simulink model "zhi_xian_er_jie_dao_li_bai"  (R2024a)
settings: Solver=VariableStepAuto  StartTime=0.0  StopTime=10.0  RelTol=1e-3
values from neighbouring files (symbols this model uses):
  epsilon = 100    [Parameters_SecondOrder_daolibai.m]
  k1 = 31.6228    [Parameters_SecondOrder_daolibai.m]
  K12 = 3/2 *(-2*m1-4*m2-4*m3)*g/((-4*m1-3*m2-12*m3)*l1)    (= 34.1214574899)    [Parameters_SecondOrder_daolibai.m]
  K12n = 3/2 *(-2*m1n-4*m2n-4*m3n)*g/((-4*m1n-3*m2n-12*m3n)*l1n)    (= 51.1821862348)    [Parameters_SecondOrder_daolibai.m]
  K13 = 9/2 * (m2*g)/((-4*m1-3*m2-12*m3)*l1)    (= -1.19028340081)    [Parameters_SecondOrder_daolibai.m]
  K13n = 9/2 * (m2n*g)/((-4*m1n-3*m2n-12*m3n)*l1n)    (= -1.78542510121)    [Parameters_SecondOrder_daolibai.m]
  K17 = 3/2*(-2*m1-m2-4*m3)/((-4*m1-3*m2-12*m3)*l1)    (= 3.36032388664)    [Parameters_SecondOrder_daolibai.m]
  K17n = 3/2*(-2*m1n-m2n-4*m3n)/((-4*m1n-3*m2n-12*m3n)*l1n)    (= 5.04048582996)    [Parameters_SecondOrder_daolibai.m]
  k2 = 200.8741    [Parameters_SecondOrder_daolibai.m]
  K22 = 2*g*(m1+2*(m2+m3))/(4*m2*l2-16/9*l2*(m1+3*(m2+m3)))    (= -63.9777327935)    [Parameters_SecondOrder_daolibai.m]
  K22n = 2*g*(m1n+2*(m2n+m3n))/(4*m2n*l2n-16/9*l2n*(m1n+3*(m2n+m3n)))    (= -76.7732793522)    [Parameters_SecondOrder_daolibai.m]
  K23 = -4/3*g*(m1+3*(m2+m3))/(4*m2*l2-16/9*l2*(m1+3*(m2+m3)))    (= 63.4817813765)    [Parameters_SecondOrder_daolibai.m]
  K23n = -4/3*g*(m1n+3*(m2n+m3n))/(4*m2n*l2n-16/9*l2n*(m1n+3*(m2n+m3n)))    (= 76.1781376518)    [Parameters_SecondOrder_daolibai.m]
  K27 = (2*(m1+2*(m2+m3))-4/3*(m1+3*(m2+m3)))/(4*m2*l2-16/9*l2*(m1+3*(m2+m3)))    (= -0.0506072874494)    [Parameters_SecondOrder_daolibai.m]
  K27n = (2*(m1n+2*(m2n+m3n))-4/3*(m1n+3*(m2n+m3n)))/(4*m2n*l2n-16/9*l2n*(m1n+3*(m2n+m3n)))    (= -0.0607287449393)    [Parameters_SecondOrder_daolibai.m]
  k3 = -315.0325    [Parameters_SecondOrder_daolibai.m]
  k4 = 28.4588    [Parameters_SecondOrder_daolibai.m]
  k5 = 3.6153    [Parameters_SecondOrder_daolibai.m]
  k6 = -36.2950    (= -36.295)    [Parameters_SecondOrder_daolibai.m]
  k_epsilon = 1    [Parameters_SecondOrder_daolibai.m]
  k_k = 1    [Parameters_SecondOrder_daolibai.m]
  k_mici = 1    [Parameters_SecondOrder_daolibai.m]
  Kd1_STC = 1    [Parameters_SecondOrder_daolibai.m]
  Kd2_STC = 1    [Parameters_SecondOrder_daolibai.m]
  u_down_limit = -200    [Parameters_SecondOrder_daolibai.m]
  u_up_limit = 200    [Parameters_SecondOrder_daolibai.m]
  x1_init = 1    [Parameters_SecondOrder_daolibai.m]
  x1_ref = 1.5    [Parameters_SecondOrder_daolibai.m]
  x2_init = 1    [Parameters_SecondOrder_daolibai.m]
  x2_ref = 0    [Parameters_SecondOrder_daolibai.m]
  x3_init = 1    [Parameters_SecondOrder_daolibai.m]
  x3_ref = 0    [Parameters_SecondOrder_daolibai.m]
  x4_init = 1    [Parameters_SecondOrder_daolibai.m]
  x5_init = 1    [Parameters_SecondOrder_daolibai.m]
  x6_init = 1    [Parameters_SecondOrder_daolibai.m]
settings Model: Creator=XieXW  LastModifiedBy=XieXW
settings SolverCC: ZeroCrossAlgorithm=Adaptive
settings DataIOCC: Refine=3
settings DebuggingCC: IgnoredZcDiagnostic=none

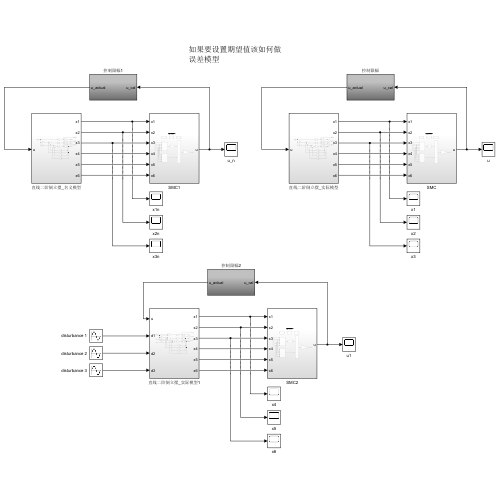
[thumbnail: Simulink's stored preview of the top-level diagram]
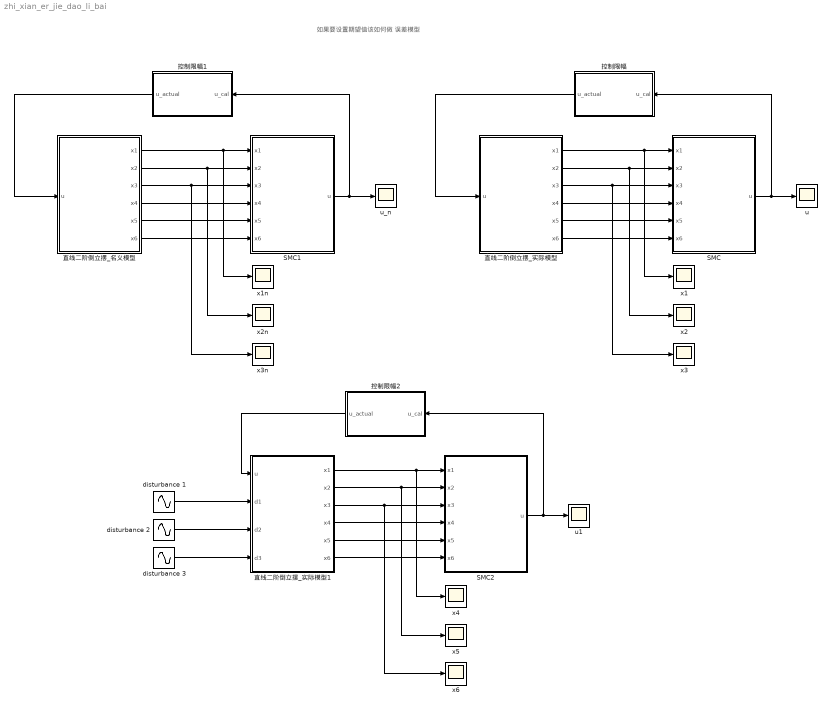
== system zhi_xian_er_jie_dao_li_bai ==
  note: 如果要设置期望值该如何做
      | 误差模型
  SMC : Subsystem
  SMC1 : Subsystem
  SMC2 : Subsystem
  disturbance 1 : Sin  Amplitude=0.05  Bias=0.1  Frequency=10  SampleTime=0
  disturbance 2 : Sin  Amplitude=0.003  Bias=0.1  Frequency=7  SampleTime=0
  disturbance 3 : Sin  Amplitude=0  Frequency=0  SampleTime=0
  u : Scope
  u1 : Scope
  u_n : Scope
  x{1..6} (6 alike) : Scope
  x1n : Scope
  x2n : Scope
  x3n : Scope
  控制限幅 : Subsystem
  控制限幅1 : Subsystem
  控制限幅2 : Subsystem
  直线二阶倒立摆_名义模型 : Subsystem
  直线二阶倒立摆_实际模型 : Subsystem
  直线二阶倒立摆_实际模型1 : Subsystem
  wires:
  直线二阶倒立摆_实际模型/1(x1) -> x1/1, SMC/1(x1)
  直线二阶倒立摆_实际模型/2(x2) -> x2/1, SMC/2(x2)
  直线二阶倒立摆_实际模型/3(x3) -> x3/1, SMC/3(x3)
  直线二阶倒立摆_实际模型/4(x4) -> SMC/4(x4)
  直线二阶倒立摆_实际模型/5(x5) -> SMC/5(x5)
  直线二阶倒立摆_实际模型/6(x6) -> SMC/6(x6)
  SMC/1(u) -> u/1, 控制限幅/1(u_cal)
  控制限幅/1(u_actual) -> 直线二阶倒立摆_实际模型/1(u)
  直线二阶倒立摆_名义模型/3(x3) -> x3n/1, SMC1/3(x3)
  SMC1/1(u) -> u_n/1, 控制限幅1/1(u_cal)
  直线二阶倒立摆_名义模型/2(x2) -> x2n/1, SMC1/2(x2)
  直线二阶倒立摆_名义模型/6(x6) -> SMC1/6(x6)
  直线二阶倒立摆_名义模型/1(x1) -> x1n/1, SMC1/1(x1)
  直线二阶倒立摆_名义模型/4(x4) -> SMC1/4(x4)
  直线二阶倒立摆_名义模型/5(x5) -> SMC1/5(x5)
  控制限幅1/1(u_actual) -> 直线二阶倒立摆_名义模型/1(u)
  直线二阶倒立摆_实际模型1/3(x3) -> x6/1, SMC2/3(x3)
  SMC2/1(u) -> u1/1, 控制限幅2/1(u_cal)
  直线二阶倒立摆_实际模型1/2(x2) -> x5/1, SMC2/2(x2)
  直线二阶倒立摆_实际模型1/6(x6) -> SMC2/6(x6)
  直线二阶倒立摆_实际模型1/1(x1) -> x4/1, SMC2/1(x1)
  直线二阶倒立摆_实际模型1/4(x4) -> SMC2/4(x4)
  直线二阶倒立摆_实际模型1/5(x5) -> SMC2/5(x5)
  控制限幅2/1(u_actual) -> 直线二阶倒立摆_实际模型1/1(u)
  disturbance 1/1 -> 直线二阶倒立摆_实际模型1/2(d1)
  disturbance 2/1 -> 直线二阶倒立摆_实际模型1/3(d2)
  disturbance 3/1 -> 直线二阶倒立摆_实际模型1/4(d3)

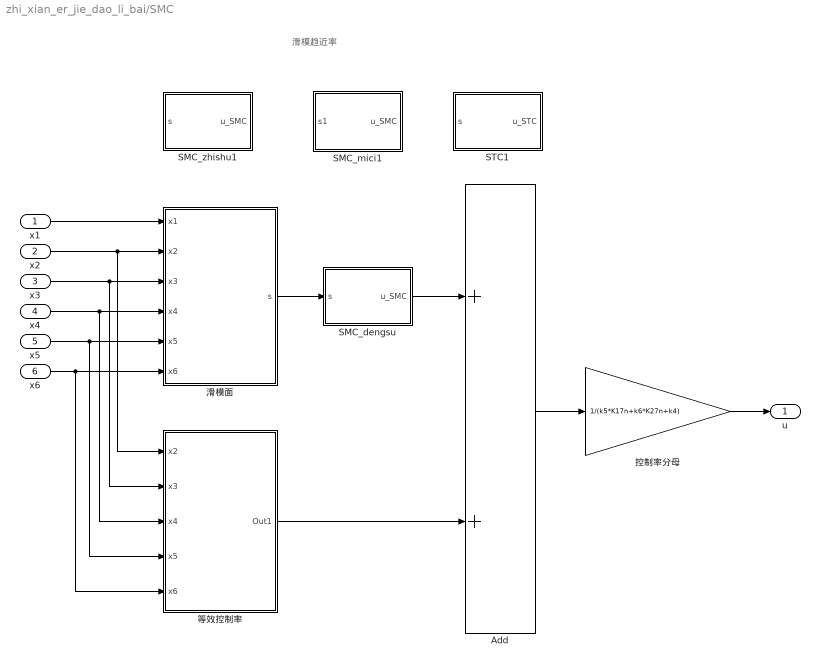
== system zhi_xian_er_jie_dao_li_bai/SMC ==
  note: 滑模趋近率
  x1 : Inport
  x2 : Inport  Port=2
  x3 : Inport  Port=3
  x4 : Inport  Port=4
  x5 : Inport  Port=5
  x6 : Inport  Port=6
  Add : Sum
  SMC_dengsu : Subsystem
  SMC_mici1 : Subsystem
  SMC_zhishu1 : Subsystem
  STC1 : Subsystem
  控制率分母 : Gain  Gain=1/(k5*K17n+k6*K27n+k4)
  滑模面 : Subsystem
  等效控制率 : Subsystem
  u : Outport
  wires:
  x1/1 -> 滑模面/1(x1)
  x2/1 -> 滑模面/2(x2), 等效控制率/1(x2)
  x3/1 -> 滑模面/3(x3), 等效控制率/2(x3)
  x4/1 -> 滑模面/4(x4), 等效控制率/3(x4)
  x5/1 -> 滑模面/5(x5), 等效控制率/4(x5)
  x6/1 -> 滑模面/6(x6), 等效控制率/5(x6)
  滑模面/1(s) -> SMC_dengsu/1(s)
  SMC_dengsu/1("u_SMC ") -> Add/1
  等效控制率/1(Out1) -> Add/2
  Add/1 -> 控制率分母/1
  控制率分母/1 -> u/1

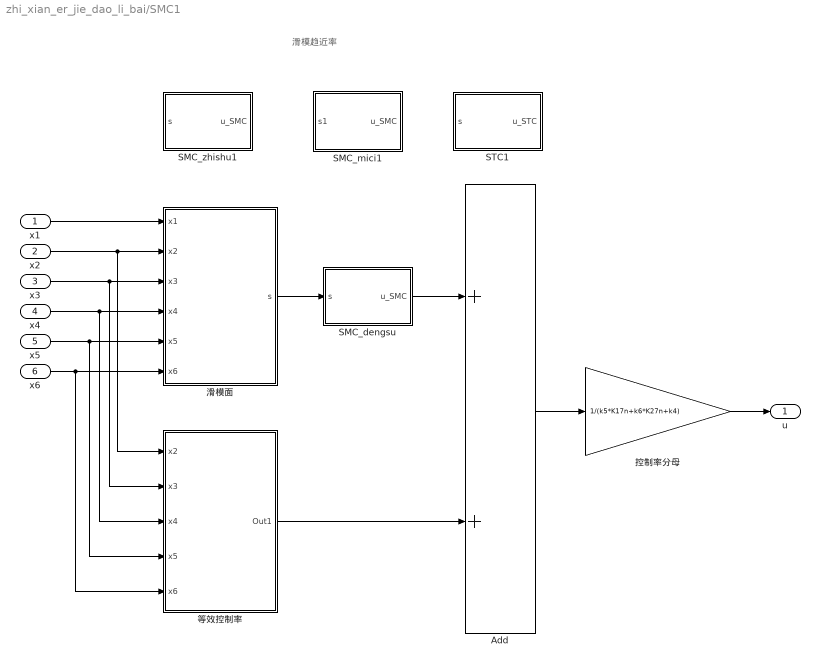
== system zhi_xian_er_jie_dao_li_bai/SMC1 ==
  note: 滑模趋近率
  x1 : Inport
  x2 : Inport  Port=2
  x3 : Inport  Port=3
  x4 : Inport  Port=4
  x5 : Inport  Port=5
  x6 : Inport  Port=6
  Add : Sum
  SMC_dengsu : Subsystem
  SMC_mici1 : Subsystem
  SMC_zhishu1 : Subsystem
  STC1 : Subsystem
  控制率分母 : Gain  Gain=1/(k5*K17n+k6*K27n+k4)
  滑模面 : Subsystem
  等效控制率 : Subsystem
  u : Outport
  wires:
  x1/1 -> 滑模面/1(x1)
  x2/1 -> 滑模面/2(x2), 等效控制率/1(x2)
  x3/1 -> 滑模面/3(x3), 等效控制率/2(x3)
  x4/1 -> 滑模面/4(x4), 等效控制率/3(x4)
  x5/1 -> 滑模面/5(x5), 等效控制率/4(x5)
  x6/1 -> 滑模面/6(x6), 等效控制率/5(x6)
  滑模面/1(s) -> SMC_dengsu/1(s)
  SMC_dengsu/1("u_SMC ") -> Add/1
  等效控制率/1(Out1) -> Add/2
  Add/1 -> 控制率分母/1
  控制率分母/1 -> u/1

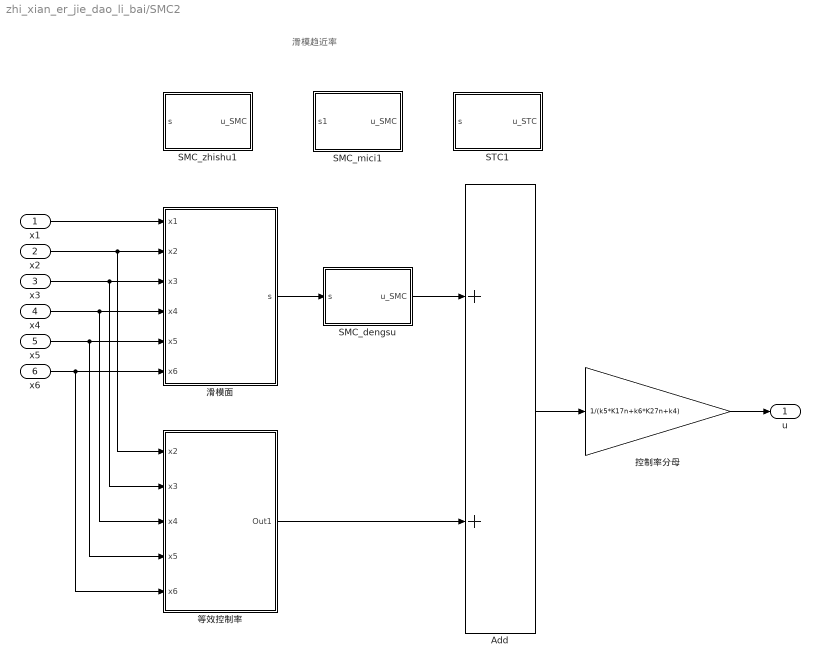
== system zhi_xian_er_jie_dao_li_bai/SMC2 ==
  note: 滑模趋近率
  x1 : Inport
  x2 : Inport  Port=2
  x3 : Inport  Port=3
  x4 : Inport  Port=4
  x5 : Inport  Port=5
  x6 : Inport  Port=6
  Add : Sum
  SMC_dengsu : Subsystem
  SMC_mici1 : Subsystem
  SMC_zhishu1 : Subsystem
  STC1 : Subsystem
  控制率分母 : Gain  Gain=1/(k5*K17n+k6*K27n+k4)
  滑模面 : Subsystem
  等效控制率 : Subsystem
  u : Outport
  wires:
  x1/1 -> 滑模面/1(x1)
  x2/1 -> 滑模面/2(x2), 等效控制率/1(x2)
  x3/1 -> 滑模面/3(x3), 等效控制率/2(x3)
  x4/1 -> 滑模面/4(x4), 等效控制率/3(x4)
  x5/1 -> 滑模面/5(x5), 等效控制率/4(x5)
  x6/1 -> 滑模面/6(x6), 等效控制率/5(x6)
  滑模面/1(s) -> SMC_dengsu/1(s)
  SMC_dengsu/1("u_SMC ") -> Add/1
  等效控制率/1(Out1) -> Add/2
  Add/1 -> 控制率分母/1
  控制率分母/1 -> u/1

== system zhi_xian_er_jie_dao_li_bai/控制限幅 ==
  u_cal : Inport
  Saturation : Saturate  UpperLimit=u_up_limit  LowerLimit=u_down_limit
  u_actual : Outport
  wires:
  u_cal/1 -> Saturation/1
  Saturation/1 -> u_actual/1

== system zhi_xian_er_jie_dao_li_bai/控制限幅1 ==
  u_cal : Inport
  Saturation : Saturate  UpperLimit=u_up_limit  LowerLimit=u_down_limit
  u_actual : Outport
  wires:
  u_cal/1 -> Saturation/1
  Saturation/1 -> u_actual/1

== system zhi_xian_er_jie_dao_li_bai/控制限幅2 ==
  u_cal : Inport
  Saturation : Saturate  UpperLimit=u_up_limit  LowerLimit=u_down_limit
  u_actual : Outport
  wires:
  u_cal/1 -> Saturation/1
  Saturation/1 -> u_actual/1

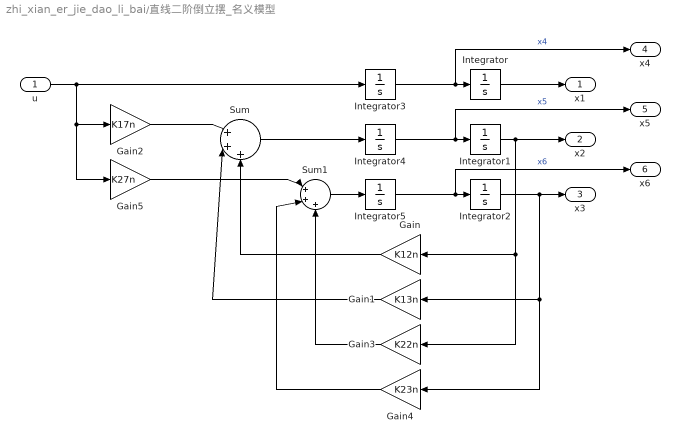
== system zhi_xian_er_jie_dao_li_bai/直线二阶倒立摆_名义模型 ==
  u : Inport
  Gain : Gain  Gain=K12n
  Gain1 : Gain  Gain=K13n
  Gain2 : Gain  Gain=K17n
  Gain3 : Gain  Gain=K22n
  Gain4 : Gain  Gain=K23n
  Gain5 : Gain  Gain=K27n
  Integrator : Integrator  InitialCondition=x1_init
  Integrator1 : Integrator  InitialCondition=x2_init
  Integrator2 : Integrator  InitialCondition=x3_init
  Integrator3 : Integrator  InitialCondition=x4_init
  Integrator4 : Integrator  InitialCondition=x5_init
  Integrator5 : Integrator  InitialCondition=x6_init
  Sum : Sum  Inputs=|+++
  Sum1 : Sum  Inputs=|+++
  x1 : Outport
  x2 : Outport  Port=2
  x3 : Outport  Port=3
  x4 : Outport  Port=4
  x5 : Outport  Port=5
  x6 : Outport  Port=6
  wires:
  Integrator/1 -> x1/1
  Integrator3/1 -> x4/1, Integrator/1  "x4"
  Integrator1/1 -> x2/1, Gain/1, Gain3/1
  Integrator2/1 -> Gain1/1, Gain4/1, x3/1
  Integrator4/1 -> x5/1, Integrator1/1  "x5"
  Integrator5/1 -> x6/1, Integrator2/1  "x6"
  u/1 -> Integrator3/1, Gain5/1, Gain2/1
  Gain/1 -> Sum/3
  Gain2/1 -> Sum/1
  Sum/1 -> Integrator4/1
  Gain1/1 -> Sum/2
  Sum1/1 -> Integrator5/1
  Gain5/1 -> Sum1/1
  Gain3/1 -> Sum1/3
  Gain4/1 -> Sum1/2

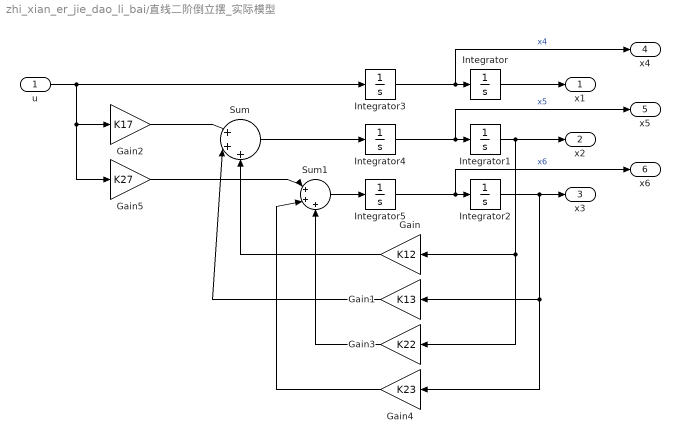
== system zhi_xian_er_jie_dao_li_bai/直线二阶倒立摆_实际模型 ==
  u : Inport
  Gain : Gain  Gain=K12
  Gain1 : Gain  Gain=K13
  Gain2 : Gain  Gain=K17
  Gain3 : Gain  Gain=K22
  Gain4 : Gain  Gain=K23
  Gain5 : Gain  Gain=K27
  Integrator : Integrator  InitialCondition=x1_init
  Integrator1 : Integrator  InitialCondition=x2_init
  Integrator2 : Integrator  InitialCondition=x3_init
  Integrator3 : Integrator  InitialCondition=x4_init
  Integrator4 : Integrator  InitialCondition=x5_init
  Integrator5 : Integrator  InitialCondition=x6_init
  Sum : Sum  Inputs=|+++
  Sum1 : Sum  Inputs=|+++
  x1 : Outport
  x2 : Outport  Port=2
  x3 : Outport  Port=3
  x4 : Outport  Port=4
  x5 : Outport  Port=5
  x6 : Outport  Port=6
  wires:
  Integrator/1 -> x1/1
  Integrator3/1 -> x4/1, Integrator/1  "x4"
  Integrator1/1 -> x2/1, Gain/1, Gain3/1
  Integrator2/1 -> Gain1/1, Gain4/1, x3/1
  Integrator4/1 -> x5/1, Integrator1/1  "x5"
  Integrator5/1 -> x6/1, Integrator2/1  "x6"
  u/1 -> Integrator3/1, Gain5/1, Gain2/1
  Gain/1 -> Sum/3
  Gain2/1 -> Sum/1
  Sum/1 -> Integrator4/1
  Gain1/1 -> Sum/2
  Sum1/1 -> Integrator5/1
  Gain5/1 -> Sum1/1
  Gain3/1 -> Sum1/3
  Gain4/1 -> Sum1/2

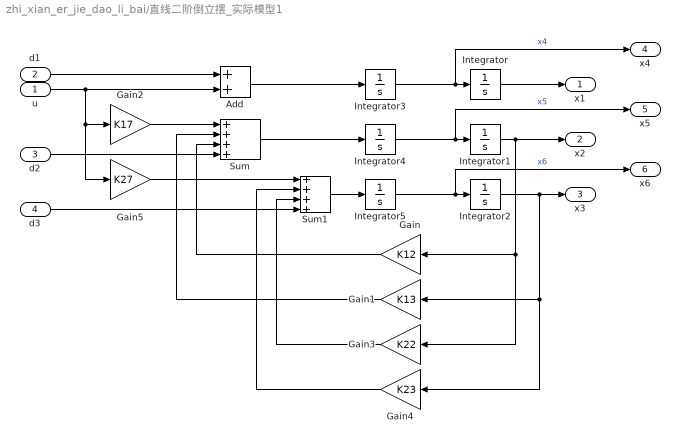
== system zhi_xian_er_jie_dao_li_bai/直线二阶倒立摆_实际模型1 ==
  u : Inport
  d1 : Inport  Port=2
  d2 : Inport  Port=3
  d3 : Inport  Port=4
  Add : Sum
  Gain : Gain  Gain=K12
  Gain1 : Gain  Gain=K13
  Gain2 : Gain  Gain=K17
  Gain3 : Gain  Gain=K22
  Gain4 : Gain  Gain=K23
  Gain5 : Gain  Gain=K27
  Integrator : Integrator  InitialCondition=x1_init
  Integrator1 : Integrator  InitialCondition=x2_init
  Integrator2 : Integrator  InitialCondition=x3_init
  Integrator3 : Integrator  InitialCondition=x4_init
  Integrator4 : Integrator  InitialCondition=x5_init
  Integrator5 : Integrator  InitialCondition=x6_init
  Sum : Sum  Inputs=++++
  Sum1 : Sum  Inputs=++++
  x1 : Outport
  x2 : Outport  Port=2
  x3 : Outport  Port=3
  x4 : Outport  Port=4
  x5 : Outport  Port=5
  x6 : Outport  Port=6
  wires:
  Integrator/1 -> x1/1
  Integrator3/1 -> x4/1, Integrator/1  "x4"
  Integrator1/1 -> x2/1, Gain/1, Gain3/1
  Integrator2/1 -> Gain1/1, Gain4/1, x3/1
  Integrator4/1 -> x5/1, Integrator1/1  "x5"
  Integrator5/1 -> x6/1, Integrator2/1  "x6"
  Gain/1 -> Sum/3
  Gain2/1 -> Sum/1
  Sum/1 -> Integrator4/1
  Gain1/1 -> Sum/2
  Sum1/1 -> Integrator5/1
  Gain5/1 -> Sum1/1
  Gain3/1 -> Sum1/3
  Gain4/1 -> Sum1/2
  Add/1 -> Integrator3/1
  d1/1 -> Add/1
  u/1 -> Gain5/1, Gain2/1, Add/2
  d2/1 -> Sum/4
  d3/1 -> Sum1/4

== system zhi_xian_er_jie_dao_li_bai/SMC/SMC_dengsu ==
  s : Inport
  Gain : Gain  Gain=epsilon
  Gain2 : Gain  Gain=-1
  Sign : Signum
  "u_SMC " : Outport
  wires:
  Gain2/1 -> "u_SMC "/1
  Gain/1 -> Gain2/1
  s/1 -> Sign/1
  Sign/1 -> Gain/1

== system zhi_xian_er_jie_dao_li_bai/SMC/SMC_mici1 ==
  s1 : Inport
  Abs : Abs  SaturateOnIntegerOverflow=off
  Gain3 : Gain  Gain=k_mici
  Gain4 : Gain  Gain=-1
  Product : Product
  Sign1 : Signum
  Sqrt : Sqrt
  "u_SMC " : Outport
  wires:
  Gain4/1 -> "u_SMC "/1
  Sign1/1 -> Product/1
  s1/1 -> Abs/1, Sign1/1
  Product/1 -> Gain3/1
  Sqrt/1 -> Product/2
  Abs/1 -> Sqrt/1
  Gain3/1 -> Gain4/1

== system zhi_xian_er_jie_dao_li_bai/SMC/SMC_zhishu1 ==
  s : Inport
  Add : Sum
  Gain : Gain  Gain=k_epsilon
  Gain1 : Gain  Gain=k_k
  Gain2 : Gain  Gain=-1
  Sign : Signum
  "u_SMC " : Outport
  wires:
  Gain2/1 -> "u_SMC "/1
  Gain1/1 -> Add/2
  Gain/1 -> Add/1
  Add/1 -> Gain2/1
  Sign/1 -> Gain/1
  s/1 -> Sign/1, Gain1/1

== system zhi_xian_er_jie_dao_li_bai/SMC/STC1 ==
  s : Inport
  Abs : Abs  SaturateOnIntegerOverflow=off
  Add : Sum
  Gain : Gain  Gain=Kd2_STC
  Gain1 : Gain  Gain=Kd1_STC
  Gain2 : Gain  Gain=-1
  Integrator : Integrator  InitialCondition=0.01
  Product : Product
  Sign : Signum
  Sqrt : Sqrt
  "u_STC " : Outport
  wires:
  Gain2/1 -> "u_STC "/1
  Add/1 -> Gain2/1
  Integrator/1 -> Gain/1
  Gain/1 -> Add/1
  Gain1/1 -> Add/2
  s/1 -> Abs/1, Sign/1
  Sqrt/1 -> Product/2
  Abs/1 -> Sqrt/1
  Product/1 -> Gain1/1
  Sign/1 -> Integrator/1, Product/1

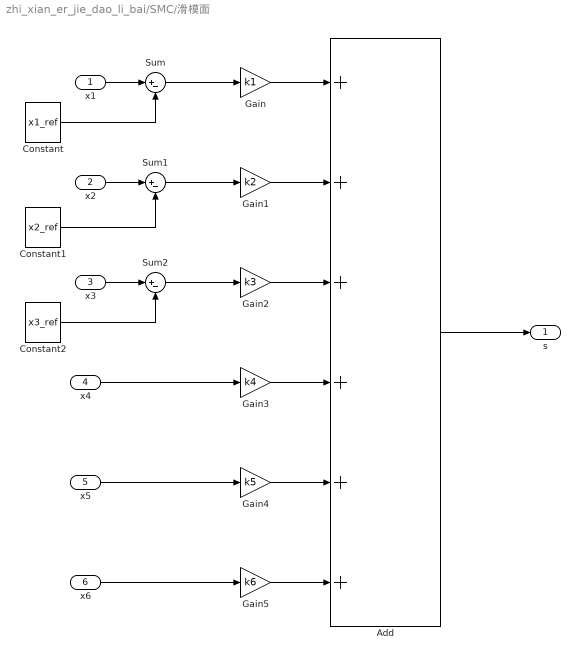
== system zhi_xian_er_jie_dao_li_bai/SMC/滑模面 ==
  x1 : Inport
  x2 : Inport  Port=2
  x3 : Inport  Port=3
  x4 : Inport  Port=4
  x5 : Inport  Port=5
  x6 : Inport  Port=6
  Add : Sum  Inputs=++++++
  Constant : Constant  Value=x1_ref
  Constant1 : Constant  Value=x2_ref
  Constant2 : Constant  Value=x3_ref
  Gain : Gain  Gain=k1
  Gain1 : Gain  Gain=k2
  Gain2 : Gain  Gain=k3
  Gain3 : Gain  Gain=k4
  Gain4 : Gain  Gain=k5
  Gain5 : Gain  Gain=k6
  Sum : Sum  Inputs=|+-
  Sum1 : Sum  Inputs=|+-
  Sum2 : Sum  Inputs=|+-
  s : Outport
  wires:
  Sum/1 -> Gain/1
  x1/1 -> Sum/1
  Constant/1 -> Sum/2
  x2/1 -> Sum1/1
  Constant1/1 -> Sum1/2
  x3/1 -> Sum2/1
  Constant2/1 -> Sum2/2
  Sum1/1 -> Gain1/1
  Sum2/1 -> Gain2/1
  x4/1 -> Gain3/1
  x5/1 -> Gain4/1
  x6/1 -> Gain5/1
  Add/1 -> s/1
  Gain/1 -> Add/1
  Gain1/1 -> Add/2
  Gain2/1 -> Add/3
  Gain3/1 -> Add/4
  Gain4/1 -> Add/5
  Gain5/1 -> Add/6

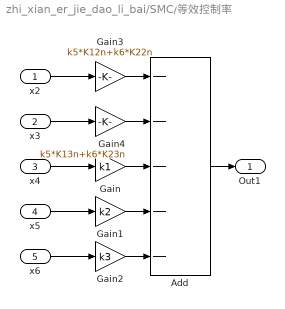
== system zhi_xian_er_jie_dao_li_bai/SMC/等效控制率 ==
  x2 : Inport
  x3 : Inport  Port=2
  x4 : Inport  Port=3
  x5 : Inport  Port=4
  x6 : Inport  Port=5
  Add : Sum  Inputs=-----
  Gain : Gain  Gain=k1
  Gain1 : Gain  Gain=k2
  Gain2 : Gain  Gain=k3
  Gain3 : Gain  Gain=k5*K12n+k6*K22n
  Gain4 : Gain  Gain=k5*K13n+k6*K23n
  Out1 : Outport
  wires:
  x4/1 -> Gain/1
  x5/1 -> Gain1/1
  x6/1 -> Gain2/1
  x2/1 -> Gain3/1
  x3/1 -> Gain4/1
  Gain2/1 -> Add/5
  Gain3/1 -> Add/1
  Gain4/1 -> Add/2
  Gain1/1 -> Add/4
  Gain/1 -> Add/3
  Add/1 -> Out1/1

== system zhi_xian_er_jie_dao_li_bai/SMC1/SMC_dengsu ==
  s : Inport
  Gain : Gain  Gain=epsilon
  Gain2 : Gain  Gain=-1
  Sign : Signum
  "u_SMC " : Outport
  wires:
  Gain2/1 -> "u_SMC "/1
  Gain/1 -> Gain2/1
  s/1 -> Sign/1
  Sign/1 -> Gain/1

== system zhi_xian_er_jie_dao_li_bai/SMC1/SMC_mici1 ==
  s1 : Inport
  Abs : Abs  SaturateOnIntegerOverflow=off
  Gain3 : Gain  Gain=k_mici
  Gain4 : Gain  Gain=-1
  Product : Product
  Sign1 : Signum
  Sqrt : Sqrt
  "u_SMC " : Outport
  wires:
  Gain4/1 -> "u_SMC "/1
  Sign1/1 -> Product/1
  s1/1 -> Abs/1, Sign1/1
  Product/1 -> Gain3/1
  Sqrt/1 -> Product/2
  Abs/1 -> Sqrt/1
  Gain3/1 -> Gain4/1

== system zhi_xian_er_jie_dao_li_bai/SMC1/SMC_zhishu1 ==
  s : Inport
  Add : Sum
  Gain : Gain  Gain=k_epsilon
  Gain1 : Gain  Gain=k_k
  Gain2 : Gain  Gain=-1
  Sign : Signum
  "u_SMC " : Outport
  wires:
  Gain2/1 -> "u_SMC "/1
  Gain1/1 -> Add/2
  Gain/1 -> Add/1
  Add/1 -> Gain2/1
  Sign/1 -> Gain/1
  s/1 -> Sign/1, Gain1/1

== system zhi_xian_er_jie_dao_li_bai/SMC1/STC1 ==
  s : Inport
  Abs : Abs  SaturateOnIntegerOverflow=off
  Add : Sum
  Gain : Gain  Gain=Kd2_STC
  Gain1 : Gain  Gain=Kd1_STC
  Gain2 : Gain  Gain=-1
  Integrator : Integrator  InitialCondition=0.01
  Product : Product
  Sign : Signum
  Sqrt : Sqrt
  "u_STC " : Outport
  wires:
  Gain2/1 -> "u_STC "/1
  Add/1 -> Gain2/1
  Integrator/1 -> Gain/1
  Gain/1 -> Add/1
  Gain1/1 -> Add/2
  s/1 -> Abs/1, Sign/1
  Sqrt/1 -> Product/2
  Abs/1 -> Sqrt/1
  Product/1 -> Gain1/1
  Sign/1 -> Integrator/1, Product/1

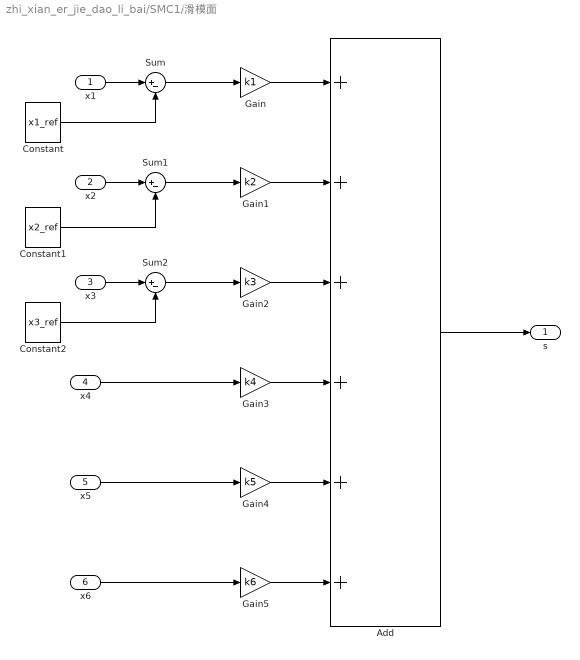
== system zhi_xian_er_jie_dao_li_bai/SMC1/滑模面 ==
  x1 : Inport
  x2 : Inport  Port=2
  x3 : Inport  Port=3
  x4 : Inport  Port=4
  x5 : Inport  Port=5
  x6 : Inport  Port=6
  Add : Sum  Inputs=++++++
  Constant : Constant  Value=x1_ref
  Constant1 : Constant  Value=x2_ref
  Constant2 : Constant  Value=x3_ref
  Gain : Gain  Gain=k1
  Gain1 : Gain  Gain=k2
  Gain2 : Gain  Gain=k3
  Gain3 : Gain  Gain=k4
  Gain4 : Gain  Gain=k5
  Gain5 : Gain  Gain=k6
  Sum : Sum  Inputs=|+-
  Sum1 : Sum  Inputs=|+-
  Sum2 : Sum  Inputs=|+-
  s : Outport
  wires:
  Sum/1 -> Gain/1
  x1/1 -> Sum/1
  Constant/1 -> Sum/2
  x2/1 -> Sum1/1
  Constant1/1 -> Sum1/2
  x3/1 -> Sum2/1
  Constant2/1 -> Sum2/2
  Sum1/1 -> Gain1/1
  Sum2/1 -> Gain2/1
  x4/1 -> Gain3/1
  x5/1 -> Gain4/1
  x6/1 -> Gain5/1
  Add/1 -> s/1
  Gain/1 -> Add/1
  Gain1/1 -> Add/2
  Gain2/1 -> Add/3
  Gain3/1 -> Add/4
  Gain4/1 -> Add/5
  Gain5/1 -> Add/6

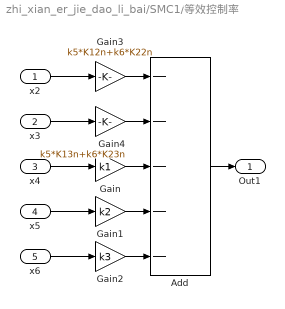
== system zhi_xian_er_jie_dao_li_bai/SMC1/等效控制率 ==
  x2 : Inport
  x3 : Inport  Port=2
  x4 : Inport  Port=3
  x5 : Inport  Port=4
  x6 : Inport  Port=5
  Add : Sum  Inputs=-----
  Gain : Gain  Gain=k1
  Gain1 : Gain  Gain=k2
  Gain2 : Gain  Gain=k3
  Gain3 : Gain  Gain=k5*K12n+k6*K22n
  Gain4 : Gain  Gain=k5*K13n+k6*K23n
  Out1 : Outport
  wires:
  x4/1 -> Gain/1
  x5/1 -> Gain1/1
  x6/1 -> Gain2/1
  x2/1 -> Gain3/1
  x3/1 -> Gain4/1
  Gain2/1 -> Add/5
  Gain3/1 -> Add/1
  Gain4/1 -> Add/2
  Gain1/1 -> Add/4
  Gain/1 -> Add/3
  Add/1 -> Out1/1

== system zhi_xian_er_jie_dao_li_bai/SMC2/SMC_dengsu ==
  s : Inport
  Gain : Gain  Gain=epsilon
  Gain2 : Gain  Gain=-1
  Sign : Signum
  "u_SMC " : Outport
  wires:
  Gain2/1 -> "u_SMC "/1
  Gain/1 -> Gain2/1
  s/1 -> Sign/1
  Sign/1 -> Gain/1

== system zhi_xian_er_jie_dao_li_bai/SMC2/SMC_mici1 ==
  s1 : Inport
  Abs : Abs  SaturateOnIntegerOverflow=off
  Gain3 : Gain  Gain=k_mici
  Gain4 : Gain  Gain=-1
  Product : Product
  Sign1 : Signum
  Sqrt : Sqrt
  "u_SMC " : Outport
  wires:
  Gain4/1 -> "u_SMC "/1
  Sign1/1 -> Product/1
  s1/1 -> Abs/1, Sign1/1
  Product/1 -> Gain3/1
  Sqrt/1 -> Product/2
  Abs/1 -> Sqrt/1
  Gain3/1 -> Gain4/1

== system zhi_xian_er_jie_dao_li_bai/SMC2/SMC_zhishu1 ==
  s : Inport
  Add : Sum
  Gain : Gain  Gain=k_epsilon
  Gain1 : Gain  Gain=k_k
  Gain2 : Gain  Gain=-1
  Sign : Signum
  "u_SMC " : Outport
  wires:
  Gain2/1 -> "u_SMC "/1
  Gain1/1 -> Add/2
  Gain/1 -> Add/1
  Add/1 -> Gain2/1
  Sign/1 -> Gain/1
  s/1 -> Sign/1, Gain1/1

== system zhi_xian_er_jie_dao_li_bai/SMC2/STC1 ==
  s : Inport
  Abs : Abs  SaturateOnIntegerOverflow=off
  Add : Sum
  Gain : Gain  Gain=Kd2_STC
  Gain1 : Gain  Gain=Kd1_STC
  Gain2 : Gain  Gain=-1
  Integrator : Integrator  InitialCondition=0.01
  Product : Product
  Sign : Signum
  Sqrt : Sqrt
  "u_STC " : Outport
  wires:
  Gain2/1 -> "u_STC "/1
  Add/1 -> Gain2/1
  Integrator/1 -> Gain/1
  Gain/1 -> Add/1
  Gain1/1 -> Add/2
  s/1 -> Abs/1, Sign/1
  Sqrt/1 -> Product/2
  Abs/1 -> Sqrt/1
  Product/1 -> Gain1/1
  Sign/1 -> Integrator/1, Product/1

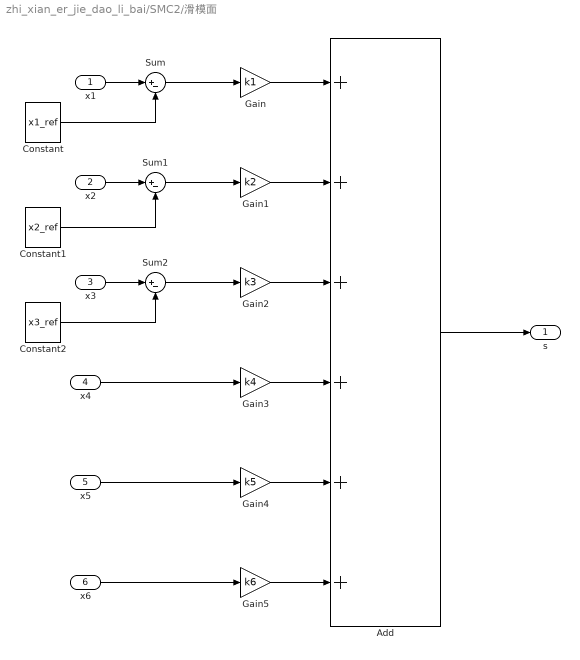
== system zhi_xian_er_jie_dao_li_bai/SMC2/滑模面 ==
  x1 : Inport
  x2 : Inport  Port=2
  x3 : Inport  Port=3
  x4 : Inport  Port=4
  x5 : Inport  Port=5
  x6 : Inport  Port=6
  Add : Sum  Inputs=++++++
  Constant : Constant  Value=x1_ref
  Constant1 : Constant  Value=x2_ref
  Constant2 : Constant  Value=x3_ref
  Gain : Gain  Gain=k1
  Gain1 : Gain  Gain=k2
  Gain2 : Gain  Gain=k3
  Gain3 : Gain  Gain=k4
  Gain4 : Gain  Gain=k5
  Gain5 : Gain  Gain=k6
  Sum : Sum  Inputs=|+-
  Sum1 : Sum  Inputs=|+-
  Sum2 : Sum  Inputs=|+-
  s : Outport
  wires:
  Sum/1 -> Gain/1
  x1/1 -> Sum/1
  Constant/1 -> Sum/2
  x2/1 -> Sum1/1
  Constant1/1 -> Sum1/2
  x3/1 -> Sum2/1
  Constant2/1 -> Sum2/2
  Sum1/1 -> Gain1/1
  Sum2/1 -> Gain2/1
  x4/1 -> Gain3/1
  x5/1 -> Gain4/1
  x6/1 -> Gain5/1
  Add/1 -> s/1
  Gain/1 -> Add/1
  Gain1/1 -> Add/2
  Gain2/1 -> Add/3
  Gain3/1 -> Add/4
  Gain4/1 -> Add/5
  Gain5/1 -> Add/6

== system zhi_xian_er_jie_dao_li_bai/SMC2/等效控制率 ==
  x2 : Inport
  x3 : Inport  Port=2
  x4 : Inport  Port=3
  x5 : Inport  Port=4
  x6 : Inport  Port=5
  Add : Sum  Inputs=-----
  Gain : Gain  Gain=k1
  Gain1 : Gain  Gain=k2
  Gain2 : Gain  Gain=k3
  Gain3 : Gain  Gain=k5*K12n+k6*K22n
  Gain4 : Gain  Gain=k5*K13n+k6*K23n
  Out1 : Outport
  wires:
  x4/1 -> Gain/1
  x5/1 -> Gain1/1
  x6/1 -> Gain2/1
  x2/1 -> Gain3/1
  x3/1 -> Gain4/1
  Gain2/1 -> Add/5
  Gain3/1 -> Add/1
  Gain4/1 -> Add/2
  Gain1/1 -> Add/4
  Gain/1 -> Add/3
  Add/1 -> Out1/1
